simulink model "test_flocking_algorithm"  (R2025b)
settings: Solver=ode4  StartTime=0.0  StopTime=200  FixedStep=0.1  RelTol=1e-3
InitFcn:
  | % initialization_2d
values from neighbouring files (symbols this model uses):
  d2r = 0.0174532925199    [DDPG_HybridFlocking_agents8-4-1.mat]    (also in flocking_learning.m; initialization_2d.m)
  g = spec(2)    [ActualOutput.m]    (also in DDPG_HybridFlocking_agents8-4-1.mat = 9.806; ModelSwarm.m; initialization.m = 9.806; initialization_2d.m = 9.806)
  m = spec(1)    [ActualOutput.m]    (also in DDPG_HybridFlocking_agents8-4-1.mat = 5; ModelSwarm.m; initialization.m = 15; initialization_2d.m = 5)
  state0 = [435.012620465 721.15936685 20 2.59881408791 0 187.945467124 786.05177403 20 2.90689824266 0 842.493878094 376.880931214 ... (25 elements, 5x5)]    [DDPG_HybridFlocking_agents8-4-1.mat]    (also in flocking_learning.m = zeros(5, N); initialization.m = [x0; y0; z0; V0; gam0; psi0]; initialization_2d.m = [x0; y0; V0; psi0; bank0])
undefined symbols (not defined in the file or in its folder): init_state
libraries: simulink_extras x10, rllib x6
(part 2 of 2)

== matlab function test_flocking_algorithm/2-Dimensional model/Subsystem/UAVs/MATLAB Function6 ==
  data: u_acs_v output; agents input; u_acs_phi output
function [u_acs_v, u_acs_phi] = ACS(agents)
    N           = size(agents, 2);
    u_acs_v     = zeros(1, N);
    u_acs_phi   = zeros(1, N);

    % Parameters
    lambda      = 1;  % CS gain
    sigma       = 1;   % ACS gain (논문의 sigma)
    beta        = 0.4;
    R           = 50;        % Desired distance
    K1          = 0.5;     % Damping
    K2          = 0.05;      % Spring
    g           = 9.806;

    if N < 2, return; end

    for i = 1:N
        %% i agent state
        pos_i       = agents(1:2, i);
        V_i         = agents(3, i);
        psi_i       = agents(4, i);
        % vel_Ni,Ei
        vel_i       = [V_i*cos(psi_i); V_i*sin(psi_i)];
        
        % Initiatializaton
        sum_acs_lon = 0;
        sum_acs_lat = 0;
        sum_cs_lon  = 0;
        sum_cs_lat  = 0;

        for j = 1:N

            if i == j, continue; end
            %% j agent state
            pos_j       = agents(1:2, j);
            V_j         = agents(3, j);
            psi_j       = agents(4, j);
            % vel_Nj,Ej
            vel_j       = [V_j*cos(psi_j); V_j*sin(psi_j)];

            rel_pos_ij = pos_i - pos_j; % (x_i - x_j)
            rel_pos_ji = pos_j - pos_i; % (x_j - x_i)
            rel_vel_ij = vel_i - vel_j; % (v_i - v_j)
            rel_vel_ji = vel_j - vel_i; % (v_j - v_i)
            r_ij        = norm(rel_pos_ij); % L2 Norm

            if r_ij < 1e-3, r_ij = 1e-3; end

            % Cucker-Smale Term (Alignment)
            eta_ij  = 1 / ((1 + r_ij^2)^beta); % communication deday rate
            % Augmented Term (Bonding Force)
            bond1   = (K1/(2*r_ij^2)) * dot(rel_vel_ij, rel_pos_ij); % damping
            bond2   = (K2/(2*r_ij)) * (r_ij - 2*R); % spring
            nu_ij   =  bond1 + bond2;

            % londitudinal force
            cs_lon  = eta_ij * (rel_vel_ji(1)*cos(psi_i) + rel_vel_ji(2)*sin(psi_i));
            acs_lon = nu_ij * (rel_pos_ji(1)*cos(psi_i) + rel_pos_ji(2)*sin(psi_i));
            % lateral force
            cs_lat  = eta_ij * (-rel_vel_ji(1)*sin(psi_i) + rel_vel_ji(2)*cos(psi_i));
            acs_lat = nu_ij * (-rel_pos_ji(1)*sin(psi_i) + rel_pos_ji(2)*cos(psi_i));

            % sum
            sum_cs_lon  = sum_cs_lon + cs_lon;
            sum_acs_lon = sum_acs_lon + acs_lon;
            sum_cs_lat  = sum_cs_lat + cs_lat;
            sum_acs_lat = sum_acs_lat + acs_lat;
        end
        % psi_dot_cmd =  (lambda/N)*sum_cs_lat; 
        % u_acs_theta(i) = (lambda/N*g)*sum_cs_lat + (sigma/N) * sum_lat; 

        u_acs_v(i)      = (lambda/N)*sum_cs_lon + (sigma/N)*sum_acs_lon;
        % u_acs_v(i)      = (sigma/N)*sum_acs_lon;
        psi_dot_cmd     = (lambda/N)*sum_cs_lat + (sigma/N)*sum_acs_lat; 
        u_acs_phi(i)    = atan2(psi_dot_cmd, g);
        % u_acs_theta(i) = 0;

    end
end

== matlab function test_flocking_algorithm/2-Dimensional model/Subsystem/MATLAB Function1 ==
  data: obs output size=9; drone_states input; psi_d input
function obs = get_observation(drone_states, psi_d)
    % drone_states: 5 x N 행렬 (x, y, z, v, psi, phi)
    % path_info: 현재 군집 중심에서 가장 가까운 경로 점 정보

    obs = zeros(9,1);
    
    % N = 10;
    v = drone_states(3, :);
    psi = drone_states(4, :);
    phi = drone_states(5, :);
    pos = drone_states(1:2, :); % x, y 위치

    % 1. VFG 지표
    center_pos = mean(pos, 2);
    R_orbit = 500;
    dist_from_origin = norm(center_pos); 
    track_error = abs(dist_from_origin - R_orbit);
    
    avg_cos = mean(cos(psi));
    avg_sin = mean(sin(psi));
    avg_psi = atan2(avg_sin, avg_cos);
    
    psi_err = psi_d - avg_psi; % Delta psi
    % obs_vfg = [track_error, sin(psi_err), cos(psi_err)];

    % 2. ACS 지표
    v_std = std(v); % O_v,std
    alignment = sqrt(avg_cos^2 + avg_sin^2); % O_align

    relative_pos = pos - center_pos; 
    all_distances = vecnorm(relative_pos, 2, 1); 

    max_dist_from_center = max(all_distances);
    % obs_acs = [v_std, alignment, max_dist_from_center];

    % 3. PF 지표
    % [PF] - 안전장치 
    dist_matrix = pdist(pos');
    if isempty(dist_matrix)
        min_dist = 1000.0; % 거리가 멀다고 가정 (충돌 방지 페널티 안 받게)
        % energy = 0.0;
    else
        min_dist = min(dist_matrix);
        % energy = 0.0;
        % a = 0.1; d_safe = 75;
        % for i = 1:length(dist_matrix)
        %     if dist_matrix(i) < d_safe
        %         energy = energy + exp(-a * (dist_matrix(i) - d_safe));
        %     end
        % end
    end
    % obs_pf = [min_dist, energy];

    % 4. Self 지표 (평균 상태)
    % obs_self = [mean(v), mean(phi)];

    % 최종 Observation 벡터 (10차원)
    % obs = [obs_vfg, obs_acs, obs_pf, obs_self]';

    s_track_error = min(track_error / 500, 1);      % 거리 오차 
    s_sin_psi     = sin(psi_err);                % 방향 오차
    s_cos_psi     = cos(psi_err);                % 방향 오차
    
    s_v_std       = min(v_std / 20, 1);          % 속도 편차 (10m/s 기준)
    s_alignment   = alignment;                    % 정렬도 (이미 0~1)
    s_max_dist    = min(max_dist_from_center / 300, 1); % 군집 반경
    s_energy_dist = (75 - min_dist) / 75;
    s_energy_dist = max(0, min(s_energy_dist, 1));

    % 최종 관측값: 제곱을 해서 거리가 가까워질수록 벌점이 기하급수적으로 커지게 함
    s_energy_mapped = s_energy_dist^2;
    % s_energy      = tanh(energy / 50);           % PF 에너지 (50단위 포화)
    
    % s_mean_v      = mean(v) / 20;                % 평균 속도 (Max 30 가정)
    % s_mean_phi    = mean(phi) / (30*180/pi);          % 평균 뱅크각 (Max 45도 가정)

    % 최종 10차원 벡터 반환
    obs = [s_track_error; s_sin_psi; s_cos_psi; s_v_std; s_alignment; ...
           s_max_dist; s_energy_mapped;  mean(v); mean(phi)];
end

== matlab function test_flocking_algorithm/2-Dimensional model/MATLAB Function3 ==
  data: all_obs output; all_states input
function all_obs = get_observation_normalized(all_states)
%% get_observation_normalized — 14차원 벡터화 관측 (k=2 nearest neighbors)
%
%  입력
%   all_states  : [5 x N]  각 열 = (x, y, V, psi, phi)
%  출력
%   all_obs     : [14 x N] 정규화된 관측
%
%  관측 채널 (각 열당 14개)
%   1)  drel_x    = (x_i - x_c)/R_form
%   2)  drel_y    = (y_i - y_c)/R_form
%   3)  dV        = (V_i - V_target)/V_target
%   4)  sin(psi_i)
%   5)  cos(psi_i)
%   6)  e_radial  = (|p_c| - R_orbit)/R_orbit
%   7)  sin(psi_des - psi_i)
%   8)  cos(psi_des - psi_i)
%   9)  Nearest 1: rel_x / R_form
%  10)  Nearest 1: rel_y / R_form
%  11)  Nearest 1: dist  / R_safe
%  12)  Nearest 2: rel_x / R_form
%  13)  Nearest 2: rel_y / R_form
%  14)  Nearest 2: dist  / R_safe
%
%  k=2 이웃 정보를 추가한 이유:
%   - 1개만 보면 "내 옆 친구가 다가오면 멀어짐" → cascade
%   - 2개 보면 "옆 친구가 다가올 때 또 다른 친구가 어디 있는지" 인식
%   - 정책이 "어느 방향으로 비키는 게 안전한지" 학습 가능
%% ------------------------------------------------------------------------

    %% 정규화 상수 (제어기 코드와 동기화)
    %  VFG: rd=500, Vd=20  /  ACS: R=50  /  PF: c=20
    R_orbit  = 500;     % VFG의 rd
    V_target = 20;      % VFG의 Vd
    R_form   = 60;      % ACS R=50 기반 + 펜타곤 여유
    R_safe   = 35;      % PF c=20 ~ ACS R=50 사이

    N       = size(all_states, 2);
    all_obs = zeros(14, N);

    pos = all_states(1:2, :);
    pc  = mean(pos, 2);

    rc       = norm(pc);
    e_radial = (rc - R_orbit) / R_orbit;
    th_c     = atan2(pc(2), pc(1));
    psi_des  = th_c + pi/2;

    for i = 1:N
        p_i   = pos(:, i);
        V_i   = all_states(3, i);
        psi_i = all_states(4, i);

        % 1,2) 중점 기준 상대 위치
        drel  = (p_i - pc) / R_form;

        % 3) 속도 오차
        dV    = (V_i - V_target) / V_target;

        % 4,5) 헤딩 sin/cos
        sP = sin(psi_i);
        cP = cos(psi_i);

        % 7,8) 접선 방향과 본인 헤딩 차이 (wrap-around 안전)
        dpsi = psi_des - psi_i;
        dpsi = atan2(sin(dpsi), cos(dpsi));
        sE   = sin(dpsi);
        cE   = cos(dpsi);

        % 9-14) 2명의 가장 가까운 이웃
        dists = inf(1, N);
        rels  = zeros(2, N);
        for j = 1:N
            if j == i, continue; end
            rel        = pos(:, j) - p_i;
            dists(j)   = norm(rel);
            rels(:, j) = rel;
        end

        % 거리 오름차순 정렬
        [sorted_d, sorted_idx] = sort(dists);

        % Nearest 1
        if sorted_d(1) < inf
            d1 = sorted_d(1);
            r1 = rels(:, sorted_idx(1));
        else
            d1 = 10 * R_safe;
            r1 = [0; 0];
        end

        % Nearest 2
        if length(sorted_d) >= 2 && sorted_d(2) < inf
            d2 = sorted_d(2);
            r2 = rels(:, sorted_idx(2));
        else
            d2 = 10 * R_safe;
            r2 = [0; 0];
        end

        obs_i = [
            drel(1); drel(2); dV; sP; cP; e_radial; sE; cE;
            r1(1)/R_form; r1(2)/R_form; d1/R_safe;
            r2(1)/R_form; r2(2)/R_form; d2/R_safe
            ];

        % 안전 클램프
        obs_i = max(min(obs_i, 10), -10);
        all_obs(:, i) = obs_i;
    end
end

== matlab function test_flocking_algorithm/2-Dimensional model/MATLAB Function4 ==
  data: all_obs input; all_rewards output; rewards_detail output
function [all_rewards, rewards_detail] = get_reward_normalized(all_obs)
%% get_reward_normalized — 음수 누적형 + Team Reward (협응 학습)
%
%  입력
%   all_obs        : [14 x N]  get_observation_normalized 출력
%
%  출력
%   all_rewards    : [1 x N]   각 에이전트 최종 보상 (개별 + 팀 mix)
%   rewards_detail : [5 x N]   세부 항목 [path; align; flock; col; surv]
%
%  보상 설계
%   r_i_individual = w_p·path_pen + w_a·align_pen + w_f·flock_pen + w_c·col_pen + surv
%   r_i_total      = 0.7 × r_i_individual + 0.3 × mean(r_individual)
%
%  Team mixing 30%의 효과:
%   - 한 명이 다른 명을 R_form 밖으로 밀어내면 자기 보상도 깎임
%   - 자연스러운 협력 압력 → cascade 방지
%   - 30% 비율은 너무 강하지 않게 (개별 학습은 70%로 유지)
%
%  관측 채널 매핑 (14차원에서 추출)
%   obs(1,2) = drel_x, drel_y     (정규화된 R_form 기준)
%   obs(6)   = e_radial           (정규화된 R_orbit 기준)
%   obs(7)   = sin(heading error)
%   obs(11)  = nearest 1 dist / R_safe
%% ------------------------------------------------------------------------

    N              = size(all_obs, 2);
    all_rewards    = zeros(1, N);
    rewards_detail = zeros(5, N);

    %% 채널별 스케일 (-10 → 0 우상향 디스플레이용)
    %  1배 스케일로 환원: episode 총합이 [-10, 0] 범위에 들어옴
    %  surv = 0 → 보상은 항상 ≤ 0, 정책 좋아지면 0에 점근
    s_path  = 0.025;
    s_align = 0.015;
    s_flock = 0.020;
    s_col   = 0.030;
    surv    = 0.0;       % 양수 항 제거 → 0을 절대 안 넘음

    %% Team Mixing 비율
    alpha_indiv = 0.7;     % 개별 보상 비중
    alpha_team  = 0.3;     % 팀 평균 보상 비중

    %% 1단계: 각 에이전트의 개별 보상 계산
    individual = zeros(1, N);
    detail     = zeros(5, N);

    for i = 1:N
        obs_i    = all_obs(:, i);
        drel_x   = obs_i(1);
        drel_y   = obs_i(2);
        e_radial = obs_i(6);
        sE       = obs_i(7);
        d_min_n  = obs_i(11);    % nearest 1 distance / R_safe

        % (1) Path error penalty
        path_pen = -s_path * e_radial^2;

        % (2) Align error penalty (heading vs path tangent)
        align_pen = -s_align * sE^2;

        % (3) Flocking penalty (R_form 바깥)
        d_norm    = sqrt(drel_x^2 + drel_y^2);
        excess    = max(0, d_norm - 1);
        flock_pen = -s_flock * excess^2;

        % (4) Collision penalty (R_safe 안)
        danger  = max(0, 1 - d_min_n);
        col_pen = -s_col * danger^2;

        % (5) Survival bonus
        surv_bonus = surv;

        total = path_pen + align_pen + flock_pen + col_pen + surv_bonus;

        % 안전 클램프
        if isnan(total) || isinf(total)
            total = -0.05;
        end
        total = max(min(total, 0), -0.05);    % per-step [-0.05, 0] (0 절대 안 넘음)

        detail(:, i)  = [path_pen; align_pen; flock_pen; col_pen; surv_bonus];
        individual(i) = total;
    end

    %% 2단계: Team Reward Mixing
    team_mean = mean(individual);

    for i = 1:N
        all_rewards(i)       = alpha_indiv * individual(i) + alpha_team * team_mean;
        rewards_detail(:, i) = detail(:, i);    % 디테일은 개별 페널티 그대로 표시
    end
end

== matlab function test_flocking_algorithm/2-Dimensional model/MATLAB Function6 ==
  data: all_states input; isdone output
function isdone = check_termination(all_states)
%% check_termination — 벡터화 종료 조건 함수
%  입력
%   all_states : [5 x N]  (x, y, V, psi, phi)
%  출력
%   isdone     : [1 x N]  1 = 해당 에이전트 종료, 0 = 계속
%
%  종료 조건 (어떤 에이전트라도 만족 시 전체 episode 종료)
%   1) 위치가 작업 영역(5km) 밖으로 이탈
%   2) 상태에 NaN/Inf 발생 (수치 폭주)
%   3) 속도가 비정상 범위 (V < 1 m/s 또는 V > 100 m/s)
%
%  Note: 충돌은 종료 조건에 포함하지 않음
%        (보상 함수의 col_pen 으로 연속적으로 학습 신호 부여)
%        → 충돌마다 episode가 끝나면 학습 데이터가 너무 적어짐
%% ------------------------------------------------------------------------

    N      = size(all_states, 2);
    isdone = false(1, N);

    %% 1) 위치 이탈
    pos = all_states(1:2, :);
    out_of_bounds = false;
    for i = 1:N
        if norm(pos(:, i)) > 5000
            out_of_bounds = true;
        end
    end

    %% 2) 수치 폭주
    nan_state = any(any(isnan(all_states))) || any(any(isinf(all_states)));

    %% 3) 비정상 속도
    V    = all_states(3, :);
    bad_V = any(V < 1) || any(V > 100);

    %% 어떤 조건이든 만족 시 모든 에이전트 종료
    if out_of_bounds || nan_state || bad_V
        isdone(:) = true;
    end
end

== matlab function test_flocking_algorithm/2-Dimensional model/UAVs/  ==
  data: u_act input; state_dot output; state input; spec input; tau input
function state_dot = ModelSwarm(u_act,state, spec, tau)
    d2r = pi/180;
    N = size(state, 2); 
    state_dot = zeros(5, N); % 초기화 스크립트와 맞춰 5행으로 설정 (x, y, V, psi, theta)
    
    g = spec(2); % 중력가속도
    
    % 시상수(Time constant) 추출
    V_tau     = tau(1);
    phi_tau = tau(2);

    for i = 1:N
        % 입력 u = [V_cmd; theta_cmd]
        V_cmd     = u_act(1, i);  % i_cat 오타 수정
        V_cmd = max(min(V_cmd, 30), 10); % 속도 제한 (10~30m/s)
        phi_cmd = u_act(2, i);  % theta_cmd (Bank angle 명령)
        
        % 현재 상태 추출 [x; y; V; psi; theta]
        V     = state(3, i); 
        V = max(min(V, 30), 15); % 속도 제한 (10~30m/s)
        psi   = state(4, i);
        % psi = max(min(psi,180*deg2rad), -180*deg2rad);
        phi = state(5, i); % 현재 Bank angle (Roll)
        phi = max(min(phi,30*d2r), -30*d2r);
        
        
        %% Kinematics & Dynamics modeling
        x_dot     = V * cos(psi);
        y_dot     = V * sin(psi);
        
        % 속도 동역학 (1차 지연 모델)
        V_dot     = (V_cmd - V)/V_tau;
        V_dot = max(min(V_dot, 5), -5); % 가속도 제한 (m/s^2)
        
        % 헤딩 동역학 (Coordinated Turn: psi_dot = g/V * tan(roll))
        % 분모 0 방지 (V가 매우 작을 때)
        if V < 0.1, V_eff = 0.1; else, V_eff = V; end
        psi_dot   = (g / V_eff) * tan(phi);
        psi_dot = max(min(psi_dot, pi/4), -pi/4);
        
        % Bank angle 동역학 (1차 지연 모델)
        % theta_cmd와 phi가 혼용되어 사용된 것을 theta_cmd와 theta로 통일
        phi_dot = (phi_cmd - phi)/phi_tau;
        phi_dot = max(min(phi_dot, pi/3), -pi/3); % 초당 60도(pi/3) 제한

        
        state_dot(:, i) = [x_dot; y_dot; V_dot; psi_dot; phi_dot];
    end
end

== matlab function test_flocking_algorithm/2-Dimensional model/UAVs/MATLAB Function1 ==
  data: states input; obs_matrix output; psi_err input; R_err input
function obs_matrix  = observation(states, psi_err, R_err)
    % states    : (5 x 20) 행렬 (N, E, V, psi, phi)
    % target_pos: [Nt; Et] 목표 선회 지점 좌표
    % rd        : 목표 선회 반경 (Loiter radius)

    % 파라미터 설명
    % ~         = 정규화시켰다는 뜻
    % ~psi_i    = 해딩각
    % ~bar{d_k,i}    = k이웃 간의 평균 거리
    % ~d_ij,min = min_j(d_ij) + 최소 쌍방향 거리
    % ~d_ki     = 폴라 좌표계에서 가장 가까운 이웃과의 상대적 거리
    % ~d_ki     = 폴라 좌표계에서 가장 가까운 이웃과의 상대적 거리에 대한 방향각??
    % ~V_ij     = 상대적인 속도 힘
    % ~e_psi,i  = VF와 관련된 해딩각 오차
    % ~e_r,i    = VF와 관련된 선회 반경

    %%
    % 파라미터 세팅
    K = 4;
    % K: 이웃 수
    % target_pos = [0 0]';
    rd= 500; % VFG 원 반경
    N_uavs = 5;
    obs_matrix = zeros(8, N_uavs); % 8x20 관측 행렬
    
    % 정규화 파라미터
    R_acs = 75; R_safe = 3; V_max = 35;
    
    
    for i = 1:N_uavs
        % --- 주체 UAV 정보 ---
        pos_i = states(1:2, i);
        Vi = states(3, i);
        psii = states(4, i);
        
        % --- 주변 UAV 전수 조사 (j-loop) ---
        dists = zeros(1, N_uavs);
        psi_diffs = zeros(1, N_uavs);
        vel_diffs = zeros(1, N_uavs);
        
        for j = 1:N_uavs
            if i == j, dists(j) = inf; continue; end
            
            dist_ij = norm(states(1:2, j) - pos_i, 2);
            dists(j) = dist_ij;
            psi_diffs(j) = atan2(sin(states(4,j)-psii), cos(states(4,j)-psii));
            vel_diffs(j) = abs(states(3,j) - Vi);
        end
        
        % K개 최근접 이웃 추출
        [sorted_dists, idx] = sort(dists);
        K_dists = sorted_dists(1:K); % 이웃
        nearest_idx = idx(1); % 그중 가장 가까운 이웃
        
        %% --- 특징 계산 및 정규화 ---
        
        % 1. 자신의 헤딩
        psii_wrapped = wrapToPi(states(4, i));
        obs_matrix(1, i) = (psii_wrapped / pi + 1) / 2;
        
        % 2. K개 이웃 평균 거리
        % --- ell 계산 (수식 그대로) ---
        ell = (2 * R_acs * sqrt(pi)) / sqrt(N_uavs);
        % --- K개 이웃 평균 거리 (이미지 하단 수식) ---
        % d_bar_ki = (1 / (K * ell)) * sum(d_ij)
        d_bar_ki = mean(K_dists) / ell; 
        obs_matrix(2, i) = min(max(d_bar_ki, 0), 1);
        
        % 3. 최소 상대 거리 (충돌 방지용)
        d_min = min(dists);
        obs_matrix(3, i) = min(max(d_min / R_safe, 0), 1);
        
        % 4 & 5. 가장 가까운 이웃과의 상대 위치 (Polar: d, psi)
        obs_matrix(4, i) = min(max(K_dists(1) / ell, 0), 1);
        dN_ij = states(1, nearest_idx) - pos_i(1); 
        dE_ij = states(2, nearest_idx) - pos_i(2);
        psi_kij = atan2(dE_ij, dN_ij);
        obs_matrix(5, i) = (psi_kij / pi + 1) / 2;
        
        % 6. 상대 속도 크기 (VK,ij)
        obs_matrix(6, i) = min(max(vel_diffs(nearest_idx) / V_max, 0), 1);
        
        % 7 &amp; 8. Vector Field(VF) 에러 (e_psi, e_r)
        % 목표 지점까지의 현재 거리 r_i
        % ri = sqrt(sum((pos_i - target_pos).^2));
        % er_i = ri - rd; % 반경 에러
        % 
        % % 현재 위치에서의 목표 헤딩(Vector Field에 의한 계산, 예시 수식)
        % % 90도는 CW/CCW 방향에 따라 가감
        % target_psi = atan2(target_pos(2)-pos_i(2), target_pos(1)-pos_i(1)) + pi/2; 
        % e_psi_i = atan2(sin(target_psi - psii), cos(target_psi - psii));
        
        obs_matrix(7, i) = min(max((psi_err(i) / pi + 1)/2, 0) ,1); % 헤딩 에러 정규화
        obs_matrix(8, i) = min(max((R_err(i) / rd + 1)/2, 0), 1); % 반경 에러 정규화
    end



end

== matlab function test_flocking_algorithm/2-Dimensional model/UAVs/MATLAB Function2 ==
  data: state input; reward output; R_err input
function reward = fcn_Reward_Calculation(state, R_err)
    % state: 5x5 행렬 (드론 5대)
    N = 5;
    xi = state(1:2, :)'; % 위치 추출 [5x2]
    % reward = zeros(1,5);
    
    % --- 파라미터 (논문 수식 기반) ---
    % pos_target = [0, 0];
    % rd = 500;       % 목표 반경
    d_safe = 5;     % 안전 거리
    % ell = 300;      % 정규화 계수
    R_acs = 75;
    
    % 보상 가중치
    K_dist = 0.5;   % 보상 가중치 (논문에 따라 조절)
    K_err = 0.05;

    %% --- 1. r_dist 계산 (전체 쌍의 거리 합) ---
    sum_dij_normalized = 0;
    pair_count = 0;
    min_dist_all = 1e6; % 전체 중 최소 거리 (r_pen용)
    ell = (2 * R_acs * sqrt(pi)) / sqrt(N);

    for i = 1:N
        for j = i+1:N % 중복 계산 방지 (i < j 조건)
            dij = norm(xi(i, :) - xi(j, :), 2);
            sum_dij_normalized = sum_dij_normalized + (dij / ell);
            pair_count = pair_count + 1; % 이것이 결국 C(n, 2)가 됨
            
            % 전체 드론 중 가장 가까운 두 녀석의 거리 체크
            if dij < min_dist_all
                min_dist_all = dij;
            end
        end
    end
    % r_dist = K_dist * (전체 거리합 / 조합 수)
    r_dist = K_dist * (sum_dij_normalized / pair_count);

    %% --- 2. r_err 계산 (전체 위치 오차의 평균) ---
    sum_err = 0;
    for i = 1:N
        sum_err = sum_err + abs(R_err(i));
    end
    % r_err = K_err * (오차 합 / n)
    r_err = K_err * (sum_err / N);

    %% --- 3. r_pen 계산 (최소 거리가 안전거리보다 작으면 3) ---
    r_pen = 0;
    if min_dist_all < d_safe
        r_pen = 3;
    end

    % --- 최종 보상 r = -(r_dist + r_err + r_pen) ---
    % 에이전트가 하나라면 스칼라로, 여러 개라면 벡터로 반환
    reward = -(r_dist + r_err + r_pen);
end

== matlab function test_flocking_algorithm/2-Dimensional model/UAVs/MATLAB Function3 ==
  data: u_act output; agents input; psi_err output; obs_input output; prev_xy_dot_des_in input; prev_xy_dot_des_out output
function [u_act, psi_err, obs_input, prev_xy_dot_des_out]  = VFG(agents,prev_xy_dot_des_in)
    % agents: [x; y; V; psi; theta] (5 x N 행렬)
    
    % --- 설정값 ---
    N = size(agents, 2);
    dt = 0.1;
    xt = 0; yt = 0;   
    Vd = 20;          % 드론이 유지해야 할 목표 속도 (m/s)
    rd = 500;         
    g = 9.806;        
    K_vf = 0.1; % 원래 1.5  
    psi_err = zeros(1,N);
    r_err = zeros(1,N);
    % curr_xy_dot_des_out = zeros(2, N); % 다음 스텝을 위해 밖으로 내보냄
    prev_xy_dot_des_out = zeros(2, N);
    % 출력 변수 초기화 (u_act: 2 x N)
    u_act = zeros(1, N);
    % des_psi = zeros(1, N);
    % psi_err = zeros(1, N);

    for i = 1 : N
        %% 1. 현재 상태 추출
        x = agents(1,i);
        y = agents(2,i);
        V = agents(3,i);      
        psi = agents(4,i);    
        
        %% 2. Vector Field 계산 (Orbit Guidance)
        xr = x - xt;
        yr = y - yt;
        r = sqrt(xr^2 + yr^2);
        r_safe = max(r, 0.1); 
        
        term1 = r_safe^2 - rd^2;
        term2 = 2 * r_safe * rd;
        
        % Vector Field 방향 생성
        xy_dot_dir = [ (term1 * xr + term2 * yr);
                       (term1 * yr - term2 * xr) ];
        
        % 현재 시점의 목표 속도 벡터
        curr_xy_dot_des = -(Vd / (r_safe * (r_safe^2 + rd^2))) * xy_dot_dir;
        % curr_xy_dot_des = xy_dot_dir;
        
        %% 3. 목표 가속도 생성 (수치 미분)
        xy_ddot_des = (curr_xy_dot_des - prev_xy_dot_des_in(:,i)) / dt;
        
        %% 4. 목표 헤딩율(dot_psi_d) 계산
        % N,E_dot
        dot_N = curr_xy_dot_des(1);
        dot_E = curr_xy_dot_des(2);

        % N,E_ddot
        % r_dot = (xr*dot_N + yr*dot_E)/r_safe;
        % ddot_N = dot_N*(r_safe^2-rd^2) - 2*xr*r_safe*r_dot + 2*rd*(dot_E*r_safe + yr*r_dot);
        % ddot_E = dot_E*(r_safe^2-rd^2) - 2*yr*r_safe*r_dot + 2*rd*(dot_N*r_safe + xr*r_dot);
        ddot_N = xy_ddot_des(1);
        ddot_E = xy_ddot_des(2);

        % desired psi
        des_psi_i = atan2(dot_E, dot_N);
        % atan2(sin, cos) 방식이 오차 계산 시 가장 안전합니다.
        % err = atan2(sin(des_psi_i - psi), cos(des_psi_i - psi));
        psi_wrapped = atan2(sin(psi), cos(psi));
        err = des_psi_i - psi_wrapped;
        % [중요] Reddit 로직: 180도(pi)를 넘어가면 반대 방향 최단거리로 보정
        if err > pi
            err = err - 2*pi;
            elseif err < -pi
                err = err + 2*pi;
        end

        psi_err(i) = err;
        r_err(i) = r;


        % desired psi_dot
        vel_sq_safe = max(dot_N^2 + dot_E^2, 0.01); 
        dot_psi_d = (ddot_E * dot_N - dot_E * ddot_N) / vel_sq_safe;
        
        %% 6. 최종 제어 입력 생성 (u_act: 2 x N)
        % 1행: 속도 명령 (멈춰있으면 안 되므로 Vd 또는 현재 V를 넣어줍니다)

        
        % 2행: 뱅크각(Roll) 명령
        u_act(1, i) = atan2(V*(dot_psi_d + K_vf * err), g);
        
        % 결과 저장
        % des_psi(i) = des_psi_i;
        % psi_err(i) = err;
        
        % 상태 업데이트
        prev_xy_dot_des_out(:,i) = curr_xy_dot_des;
        obs_input = [xt,yt, rd]';
    end
end

== matlab function test_flocking_algorithm/2-Dimensional model/UAVs/MATLAB Function4 ==
  data: u_pf output; agents input; spec input; pf output; pf_lat output; sum_pf output
function [u_pf, pf, pf_lat, sum_pf]  = PF(agents, spec)

    %% params
    % idx = 1;
    N = size(agents,2);
    alp = 9; % Potential Strength
    % Bell Function Constant (a, b, c)
    a   = 10; 
    b   = 2;
    c   = 20;
    u_pf = zeros(1,N);
    pf = zeros(1,N);
    denominator = 0;
    sum_pf = zeros(2,N);

    g = spec(2);

    %% Algorithm
    for idx = 1: N
        pos_i = agents(1:2, idx);
        psi = agents(4, idx);
        sum = zeros(2,1);

        for j = 1: N
            if idx==j 
                continue; 
            end
            pos_j = agents(1:2, j);
            pos_ij = pos_i - pos_j;
            pos_ji = pos_j - pos_i;
            norm_ij = norm(pos_ij);
    
            val = (norm_ij - c)/a;
            denominator = 1 + val^(2*b);
            if norm_ij > 0.001
                sum = sum + (alp/denominator)*(pos_ji/norm_ij);
            end
        end
        pf_lat = [-sin(psi) cos(psi)]*[sum(1); sum(2)];
        phi_cmd = atan2(pf_lat, g);
        u_pf(1,idx) = phi_cmd;
        pf(1,idx) = denominator; 
        sum_pf(:,idx) = sum;
    end
end

== matlab function test_flocking_algorithm/2-Dimensional model/UAVs/MATLAB Function6 ==
  data: u_acs_v output; agents input; u_acs_phi output
function [u_acs_v, u_acs_phi] = ACS(agents)
    N           = size(agents, 2);
    u_acs_v     = zeros(1, N);
    u_acs_phi   = zeros(1, N);

    % Parameters
    lambda      = 0.5;  % CS gain
    sigma       = 1;   % ACS gain (논문의 sigma)
    beta        = 0.2;
    R           = 50;        % Desired distance
    K1          = 0.5;     % Damping
    K2          = 0.1;      % Spring
    g           = 9.806;

    if N < 2, return; end

    for i = 1:N
        %% i agent state
        pos_i       = agents(1:2, i);
        V_i         = agents(3, i);
        psi_i       = agents(4, i);
        % vel_Ni,Ei
        vel_i       = [V_i*cos(psi_i); V_i*sin(psi_i)];
        
        % Initiatializaton
        sum_acs_lon = 0;
        sum_acs_lat = 0;
        sum_cs_lon  = 0;
        sum_cs_lat  = 0;

        for j = 1:N

            if i == j, continue; end
            %% j agent state
            pos_j       = agents(1:2, j);
            V_j         = agents(3, j);
            psi_j       = agents(4, j);
            % vel_Nj,Ej
            vel_j       = [V_j*cos(psi_j); V_j*sin(psi_j)];

            rel_pos_ij = pos_i - pos_j; % (x_i - x_j)
            rel_pos_ji = pos_j - pos_i; % (x_j - x_i)
            rel_vel_ij = vel_i - vel_j; % (v_i - v_j)
            rel_vel_ji = vel_j - vel_i; % (v_j - v_i)
            r_ij        = norm(rel_pos_ij); % L2 Norm

            if r_ij < 1e-3, r_ij = 1e-3; end

            % Cucker-Smale Term (Alignment)
            eta_ij  = 1 / ((1 + r_ij^2)^beta); % communication deday rate
            % Augmented Term (Bonding Force)
            bond1   = (K1/(2*r_ij^2)) * dot(rel_vel_ij, rel_pos_ij); % damping
            bond2   = (K2/(2*r_ij)) * (r_ij - 2*R); % spring
            nu_ij   =  bond1 + bond2;

            % londitudinal force
            cs_lon  = eta_ij * (rel_vel_ji(1)*cos(psi_i) + rel_vel_ji(2)*sin(psi_i));
            acs_lon = nu_ij * (rel_pos_ji(1)*cos(psi_i) + rel_pos_ji(2)*sin(psi_i));
            % lateral force
            cs_lat  = eta_ij * (-rel_vel_ji(1)*sin(psi_i) + rel_vel_ji(2)*cos(psi_i));
            acs_lat = nu_ij * (-rel_pos_ji(1)*sin(psi_i) + rel_pos_ji(2)*cos(psi_i));

            % sum
            sum_cs_lon  = sum_cs_lon + cs_lon;
            sum_acs_lon = sum_acs_lon + acs_lon;
            sum_cs_lat  = sum_cs_lat + cs_lat;
            sum_acs_lat = sum_acs_lat + acs_lat;
        end
        % psi_dot_cmd =  (lambda/N)*sum_cs_lat; 
        % u_acs_theta(i) = (lambda/N*g)*sum_cs_lat + (sigma/N) * sum_lat; 

        u_acs_v(i)      = (lambda/N)*sum_cs_lon + (sigma/N)*sum_acs_lon;
        % u_acs_v(i)      = (sigma/N)*sum_acs_lon;
        psi_dot_cmd     = (lambda/N)*sum_cs_lat + (sigma/N)*sum_acs_lat; 
        u_acs_phi(i)    = atan2(psi_dot_cmd, g);
        % u_acs_theta(i) = 0;

    end
end

== matlab function test_flocking_algorithm/2-Dimensional model/Subsystem/UAVs/  ==
  data: u_act input; state_dot output; state input; spec input; tau input
function state_dot = ModelSwarm(u_act,state, spec, tau)
    d2r = pi/180;
    N = size(state, 2); 
    state_dot = zeros(5, N); % 초기화 스크립트와 맞춰 5행으로 설정 (x, y, V, psi, theta)
    
    g = spec(2); % 중력가속도
    
    % 시상수(Time constant) 추출
    V_tau     = tau(1);
    phi_tau = tau(2);

    for i = 1:N
        % 입력 u = [V_cmd; theta_cmd]
        V_cmd     = u_act(1, i);  % i_cat 오타 수정
        V_cmd = max(min(V_cmd, 30), 10); % 속도 제한 (10~30m/s)
        phi_cmd = u_act(2, i);  % theta_cmd (Bank angle 명령)
        
        % 현재 상태 추출 [x; y; V; psi; theta]
        V     = state(3, i); 
        V = max(min(V, 30), 15); % 속도 제한 (10~30m/s)
        psi   = state(4, i);
        % psi = max(min(psi,180*deg2rad), -180*deg2rad);
        phi = state(5, i); % 현재 Bank angle (Roll)
        phi = max(min(phi,30*d2r), -30*d2r);
        
        
        %% Kinematics & Dynamics modeling
        x_dot     = V * cos(psi);
        y_dot     = V * sin(psi);
        
        % 속도 동역학 (1차 지연 모델)
        V_dot     = (V_cmd - V)/V_tau;
        V_dot = max(min(V_dot, 5), -5); % 가속도 제한 (m/s^2)
        
        % 헤딩 동역학 (Coordinated Turn: psi_dot = g/V * tan(roll))
        % 분모 0 방지 (V가 매우 작을 때)
        if V < 0.1, V_eff = 0.1; else, V_eff = V; end
        psi_dot   = (g / V_eff) * tan(phi);
        psi_dot = max(min(psi_dot, pi/4), -pi/4);
        
        % Bank angle 동역학 (1차 지연 모델)
        % theta_cmd와 phi가 혼용되어 사용된 것을 theta_cmd와 theta로 통일
        phi_dot = (phi_cmd - phi)/phi_tau;
        phi_dot = max(min(phi_dot, pi/3), -pi/3); % 초당 60도(pi/3) 제한

        
        state_dot(:, i) = [x_dot; y_dot; V_dot; psi_dot; phi_dot];
    end
end

== matlab function test_flocking_algorithm/2-Dimensional model/Subsystem/UAVs/MATLAB Function1 ==
  data: states input; obs_matrix output; psi_err input; R_err input
function obs_matrix  = observation(states, psi_err, R_err)
    % states    : (5 x 20) 행렬 (N, E, V, psi, phi)
    % target_pos: [Nt; Et] 목표 선회 지점 좌표
    % rd        : 목표 선회 반경 (Loiter radius)

    % 파라미터 설명
    % ~         = 정규화시켰다는 뜻
    % ~psi_i    = 해딩각
    % ~bar{d_k,i}    = k이웃 간의 평균 거리
    % ~d_ij,min = min_j(d_ij) + 최소 쌍방향 거리
    % ~d_ki     = 폴라 좌표계에서 가장 가까운 이웃과의 상대적 거리
    % ~d_ki     = 폴라 좌표계에서 가장 가까운 이웃과의 상대적 거리에 대한 방향각??
    % ~V_ij     = 상대적인 속도 힘
    % ~e_psi,i  = VF와 관련된 해딩각 오차
    % ~e_r,i    = VF와 관련된 선회 반경

    %%
    % 파라미터 세팅
    K = 4;
    % K: 이웃 수
    % target_pos = [0 0]';
    rd= 500; % VFG 원 반경
    N_uavs = 5;
    obs_matrix = zeros(8, N_uavs); % 8x20 관측 행렬
    
    % 정규화 파라미터
    R_acs = 75; R_safe = 3; V_max = 35;
    
    
    for i = 1:N_uavs
        % --- 주체 UAV 정보 ---
        pos_i = states(1:2, i);
        Vi = states(3, i);
        psii = states(4, i);
        
        % --- 주변 UAV 전수 조사 (j-loop) ---
        dists = zeros(1, N_uavs);
        psi_diffs = zeros(1, N_uavs);
        vel_diffs = zeros(1, N_uavs);
        
        for j = 1:N_uavs
            if i == j, dists(j) = inf; continue; end
            
            dist_ij = norm(states(1:2, j) - pos_i, 2);
            dists(j) = dist_ij;
            psi_diffs(j) = atan2(sin(states(4,j)-psii), cos(states(4,j)-psii));
            vel_diffs(j) = abs(states(3,j) - Vi);
        end
        
        % K개 최근접 이웃 추출
        [sorted_dists, idx] = sort(dists);
        K_dists = sorted_dists(1:K); % 이웃
        nearest_idx = idx(1); % 그중 가장 가까운 이웃
        
        %% --- 특징 계산 및 정규화 ---
        
        % 1. 자신의 헤딩
        psii_wrapped = wrapToPi(states(4, i));
        obs_matrix(1, i) = (psii_wrapped / pi + 1) / 2;
        
        % 2. K개 이웃 평균 거리
        % --- ell 계산 (수식 그대로) ---
        ell = (2 * R_acs * sqrt(pi)) / sqrt(N_uavs);
        % --- K개 이웃 평균 거리 (이미지 하단 수식) ---
        % d_bar_ki = (1 / (K * ell)) * sum(d_ij)
        d_bar_ki = mean(K_dists) / ell; 
        obs_matrix(2, i) = min(max(d_bar_ki, 0), 1);
        
        % 3. 최소 상대 거리 (충돌 방지용)
        d_min = min(dists);
        obs_matrix(3, i) = min(max(d_min / R_safe, 0), 1);
        
        % 4 & 5. 가장 가까운 이웃과의 상대 위치 (Polar: d, psi)
        obs_matrix(4, i) = min(max(K_dists(1) / ell, 0), 1);
        dN_ij = states(1, nearest_idx) - pos_i(1); 
        dE_ij = states(2, nearest_idx) - pos_i(2);
        psi_kij = atan2(dE_ij, dN_ij);
        obs_matrix(5, i) = (psi_kij / pi + 1) / 2;
        
        % 6. 상대 속도 크기 (VK,ij)
        obs_matrix(6, i) = min(max(vel_diffs(nearest_idx) / V_max, 0), 1);
        
        % 7 &amp; 8. Vector Field(VF) 에러 (e_psi, e_r)
        % 목표 지점까지의 현재 거리 r_i
        % ri = sqrt(sum((pos_i - target_pos).^2));
        % er_i = ri - rd; % 반경 에러
        % 
        % % 현재 위치에서의 목표 헤딩(Vector Field에 의한 계산, 예시 수식)
        % % 90도는 CW/CCW 방향에 따라 가감
        % target_psi = atan2(target_pos(2)-pos_i(2), target_pos(1)-pos_i(1)) + pi/2; 
        % e_psi_i = atan2(sin(target_psi - psii), cos(target_psi - psii));
        
        obs_matrix(7, i) = min(max((psi_err(i) / pi + 1)/2, 0) ,1); % 헤딩 에러 정규화
        obs_matrix(8, i) = min(max((R_err(i) / rd + 1)/2, 0), 1); % 반경 에러 정규화
    end



end

== matlab function test_flocking_algorithm/2-Dimensional model/Subsystem/UAVs/MATLAB Function2 ==
  data: state input; reward output; R_err input
function reward = fcn_Reward_Calculation(state, R_err)
    % state: 5x5 행렬 (드론 5대)
    N = 5;
    xi = state(1:2, :)'; % 위치 추출 [5x2]
    % reward = zeros(1,5);
    
    % --- 파라미터 (논문 수식 기반) ---
    % pos_target = [0, 0];
    % rd = 500;       % 목표 반경
    d_safe = 5;     % 안전 거리
    % ell = 300;      % 정규화 계수
    R_acs = 75;
    
    % 보상 가중치
    K_dist = 0.5;   % 보상 가중치 (논문에 따라 조절)
    K_err = 0.05;

    %% --- 1. r_dist 계산 (전체 쌍의 거리 합) ---
    sum_dij_normalized = 0;
    pair_count = 0;
    min_dist_all = 1e6; % 전체 중 최소 거리 (r_pen용)
    ell = (2 * R_acs * sqrt(pi)) / sqrt(N);

    for i = 1:N
        for j = i+1:N % 중복 계산 방지 (i < j 조건)
            dij = norm(xi(i, :) - xi(j, :), 2);
            sum_dij_normalized = sum_dij_normalized + (dij / ell);
            pair_count = pair_count + 1; % 이것이 결국 C(n, 2)가 됨
            
            % 전체 드론 중 가장 가까운 두 녀석의 거리 체크
            if dij < min_dist_all
                min_dist_all = dij;
            end
        end
    end
    % r_dist = K_dist * (전체 거리합 / 조합 수)
    r_dist = K_dist * (sum_dij_normalized / pair_count);

    %% --- 2. r_err 계산 (전체 위치 오차의 평균) ---
    sum_err = 0;
    for i = 1:N
        sum_err = sum_err + abs(R_err(i));
    end
    % r_err = K_err * (오차 합 / n)
    r_err = K_err * (sum_err / N);

    %% --- 3. r_pen 계산 (최소 거리가 안전거리보다 작으면 3) ---
    r_pen = 0;
    if min_dist_all < d_safe
        r_pen = 3;
    end

    % --- 최종 보상 r = -(r_dist + r_err + r_pen) ---
    % 에이전트가 하나라면 스칼라로, 여러 개라면 벡터로 반환
    reward = -(r_dist + r_err + r_pen);
end

== matlab function test_flocking_algorithm/3-Dimensional model/ActualOutput/MATLAB Function ==
  data: u_virtual input; act_cmd output; state input; spec input
function act_cmd = ActualOutput(u_virtual, state, spec)
    % 1. 에이전트 수 인식
    N = size(state, 2);
    
    % 2. [중요] 출력 행렬 초기화
    % MATLAB에게 최대 100대까지는 감당할 수 있다고 '상한선'을 알려줍니다.
    % 시뮬레이션 환경에 따라 20, 50, 100 등 적절한 숫자를 넣으세요.
    act_cmd = zeros(3, N); 
    % 만약 spec이 [2x20]이라면 spec(1, i)로 써야 합니다.
    m = spec(1); 
    g = spec(2);
    D = 0;
    for i = 1:N
        %% Virtual Input (i번째 열 추출)
        ux = u_virtual(1, i);
        uy = u_virtual(2, i);
        uz = u_virtual(3, i);
        
        %% state (i번째 열 추출)
        gam = state(5, i); % flight path angle
        psi = state(6, i); % Heading angle
        
        %%     
        % bank angle
        num_phi     = uy * cos(psi) - ux * sin(psi);
        den_phi     = (g+uz) * cos(gam) - (ux * cos(psi) + uy * sin(psi)) * sin(gam);
        phi         = atan2(num_phi, den_phi);
        
        % Lift
        den_phi     = (g+uz) * cos(gam) - (ux * cos(psi) + uy * sin(psi)) * sin(gam);
        L           = m * (den_phi / cos(phi));
        
        % Thrust
        horz_acc    = ux * cos(psi) + uy * sin(psi);
        T           = m * ((g+uz) * sin(gam) + horz_acc * cos(gam)) + D;
        
        %% [물리적 제한] 주석 해제 추천 (시뮬레이션 폭주 방지)
        % phi = max(min(phi, pi/3), -pi/3); 
        % L   = max(L, 0); 
        % T   = max(T, 0); 
        
        % 세로 벡터(3x1)로 i번째 열에 저장
        act_cmd(:, i) = [phi; L; T]; 
    end
end

== matlab function test_flocking_algorithm/3-Dimensional model/MATLAB Function ==
  data: u_act input; state_dot output; state input; spec input
function state_dot = ModelSwarm(u_act, state, spec)
    % ut: [3 x 20] (phi, L, T 명령 행렬)
    % state: [6 x 20] (현재 20대의 상태 행렬)
    % spec_matrix: [2 x 20] (20대의 질량, 중력 행렬)

    N = size(state, 2); % 에이전트 수 자동 인식 (20대)
    state_dot = zeros(6, N); % 미분값 저장용 행렬 예약

    % 1. i번째 드론의 파라미터와 입력만 쏙 뽑기
    m = spec(1);
    g = spec(2);
    D = 0;
    
    for i = 1:N
        
        phi = u_act(1, i); 
        L = u_act(2, i); 
        T = u_act(3, i);

        V   = state(4, i); 
        gam = state(5, i); 
        psi = state(6, i);

        % 2. 기존에 만드신 1대용 물리 법칙 적용
        x_dot = V*cos(gam)*cos(psi);
        y_dot = V*cos(gam)*sin(psi);
        z_dot = -V*sin(gam);
        
        %% Dynamics
        VT_dot      = (T - D)/m - g*sin(gam);
        gam_dot     = (L*cos(phi) - m*g*cos(gam)) / (m*V+ eps);
        psi_dot     = (L*sin(phi)) / (m*V*cos(gam)+ eps);
        
        % 3. i번째 열에 결과 저장
        state_dot(:, i) = [x_dot; y_dot; z_dot; VT_dot; gam_dot; psi_dot];
    end
end

== matlab function test_flocking_algorithm/3-Dimensional model/Synthesize Commands/MATLAB Function ==
  data: u_acs output; agents input
function u_acs = ACS(agents)

    %% Agent parameters
    % idx     = 1;
    N       = size(agents,2);
    % pos_i   = agents(1:3, idx);
    % vel_i   = agents(4:6, idx);

    %% damping parameters
    K1      = 0.32; % Bonding gain 1
    % damping = zeros(3,N);

    %% spring parameters
    R       = 75;
    K2      = 0.5; % Bonding gain 2
    % spring  = zeros(3,N);

    u_acs = zeros(3,N);

    %% CS model algorithm
    lamda       = 1; % Alignment Strength
    beta        = 0.25; % Communication Decay rate

    if N < 2
        return;
    end

    %% Algorithm
    for idx = 1 : N
        % ith Position
        pos_i   = agents(1:3, idx); % Position
        % ith Velocity
        V       = agents(4,idx);
        gam_i     = agents(5,idx);
        psi_i     = agents(6,idx);
        xi_dot   = V*cos(gam_i)*cos(psi_i);
        yi_dot   = V*cos(gam_i)*sin(psi_i);
        zi_dot   = V*sin(gam_i);
        vel_i   = [xi_dot yi_dot zi_dot]'; % Velocity

        damping = zeros(3,1);
        spring  = zeros(3,1); 
        cs      = zeros(3,1);

        for j = 1 : N
            if j == idx, continue; end
            % jth Velocity
            pos_j   = agents(1:3, j);
            % jth Velocity
            V       = agents(4,j);
            gam_j   = agents(5,j);
            psi_j   = agents(6,j);
            xj_dot  = V*cos(gam_j)*cos(psi_j);
            yj_dot  = V*cos(gam_j)*sin(psi_j);
            zj_dot  = V*sin(gam_j);
            vel_j   = [xj_dot yj_dot zj_dot]'; % Velocity

            pos_ij  = pos_i - pos_j;
            pos_ji  = pos_j - pos_i;
            vel_ij  = vel_i - vel_j;

            r_ij    = norm(pos_ij);
    
            if r_ij < 1e-3, r_ij = 1e-3; end

            % communication decay rate
            com     = 1 / (1+r_ij^2)^beta;
            vel     = vel_j - vel_i;

            cs = cs + com*vel; 
            
            % Inner Product
            dot_val = dot(vel_ij, pos_ij);
            % Damping term
            damping = damping + ((K1 / (2 * r_ij^2)) * dot_val) * (pos_j - pos_i);
            
            % Spring term
            spring  = spring +  ((K2 / (2 * r_ij)) * (r_ij - 2*R)) * (pos_j - pos_i);
        end
        u_acs(:,idx) = (lamda/N)*cs + (1/N)*(damping + spring);
    end


end

== matlab function test_flocking_algorithm/3-Dimensional model/Synthesize Commands/MATLAB Function1 ==
  data: VFG output; agents input; psi output; des_psi output; psi_err output
function [VFG, psi ,des_psi, psi_err] = VFG(agents)
    N = size(agents, 2);
    VFG = zeros(3,N);
    xt = 0; yt = 0; zt = -100; % Target Position (NED 기준, -100m는 상공)
    Vd = 20;                   % Desired Speed
    rd = 500;                  % Desired Orbit Radius

    for i = 1 : N
        %% 1. State Input (Inertial Frame)
        x = agents(1,i);
        y = agents(2,i);
        z = agents(3,i);
        V = agents(4,i);      % Airspeed (or Groundspeed)
        gam = agents(5,i);    % Flight path angle
        psi = agents(6,i);    % Heading angle
        % psi = atan2(sin(psi), cos(psi));
        % des_psi = psi;
        
        %% 2. Desired Velocity Vector Field (Equation 7)
        xr = x - xt;
        yr = y - yt;
        r = sqrt(xr^2 + yr^2);
        
        % 분모 0 방지 및 수치 안정성 확보
        r_safe = max(r, 0.01);
        
        % Matrix A &amp; B formulation (Equation 7)
        % 논문의 수식: [xr(r^2-rd^2) + yr(2r rd); yr(r^2-rd^2) - xr(2r rd)]
        % A = [ (r_safe^2 - rd^2),   (2 * r_safe * rd); 
        %      -(2 * r_safe * rd),   (r_safe^2 - rd^2) ];
        % B = [xr; yr];
        
        xy_dot = [ 
            (r_safe^2 - rd^2)*xr + (2*r_safe*rd)*yr ;
            (r_safe^2 - rd^2)*yr - (2*r_safe*rd)*xr
            ];
        
        % xy_dot_des = [dot_x_di; dot_y_di]
        xy_dot_des = -(Vd / (r_safe * (r_safe^2 + rd^2))) .* xy_dot;
        
        %% 4. Desired Heading Angle (Equation 8)
        
        des_psi = atan2(xy_dot_des(2), xy_dot_des(1));
        
        psi_wrapped = atan2(sin(psi), cos(psi));
        %% 5. Control Commands in Horizontally Body-fixed Frame (Equation 5)
        
        
        % U2: Heading tracking (Lateral) - Angle Wrap-around 처리 필수
        % psi_err = des_psi - psi;
        % psi_err = atan2(sin(des_psi - psi), cos(des_psi - psi));
        
        % 목표와 현재 각도의 차이 구하기
        psi_err = des_psi - psi_wrapped;
        % [중요] Reddit 로직: 180도(pi)를 넘어가면 반대 방향 최단거리로 보정
        if psi_err > pi
            psi_err = psi_err - 2*pi;
        elseif psi_err < -pi
            psi_err = psi_err + 2*pi;
        end
        
        
        U1 = Vd - V * cos(gam); % U1: Speed tracking (Longitudinal)
        U2 = V * psi_err;
        U3 = zt - z; % U3: Altitude tracking (Vertical)
        U = [U1; U2; U3];
        
        %% 6. Transform to Inertial Frame (Equation 6)
        % R_psi rotation matrix
        tran = [
            cos(psi) -sin(psi) 0;
            sin(psi)  cos(psi) 0;
            0         0        1
            ];
        
        
        % 가속도(또는 속도 변화율) 명령 생성
        VFG(:,i) = tran * U;
    end
end

== matlab function test_flocking_algorithm/3-Dimensional model/Synthesize Commands/MATLAB Function2 ==
  data: u_pf output; agents input
function u_pf = PF(agents)

    %% params
    % idx = 1;
    N = size(agents,2);
    alp = 5*sqrt(2); % Potential Strength
    % Bell Function Constant (a, b, c)
    a   = 15; 
    b   = 4;
    c   = 10;
    u_pf = zeros(3,N);

    %% Algorithm
    for idx = 1: N
        pos_i = agents(1:3, idx);
        sum = zeros(3,1);

        for j = 1: N
            if idx==j 
                continue; 
            end
            pos_j = agents(1:3, j);
            pos_ij = pos_i - pos_j;
            norm_ij = norm(pos_ij);
    
            val = (norm_ij - c)/a;
            denominator = 1 + (abs(val))^(2*b);
            if norm_ij > 0.001
                sum = sum + (alp/denominator)*(pos_ij/norm_ij);
            end
        end
    u_pf(:,idx) = sum;
    end
end
